simulink model "WindTurbineModelFinalPMSGASTW1"  (R2024a)
settings: Solver=ode1  StartTime=0.0  StopTime=50  FixedStep=0.0001  RelTol=1e-3
InitFcn:
  | ng       = 97;
model workspace: external: MAT-File C:\Users\anif4\Downloads\Cp_Model_5thOrder.mat (data not in the file)
settings Model: Creator=user  LastModifiedBy=anif4
settings RTWCC: GPUComputeCapability=3.5

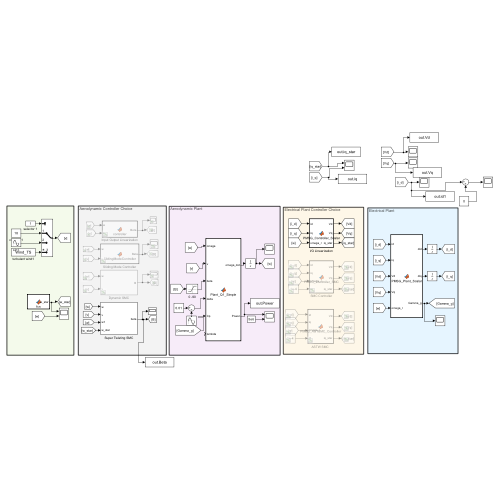
[thumbnail: Simulink's stored preview of the top-level diagram]
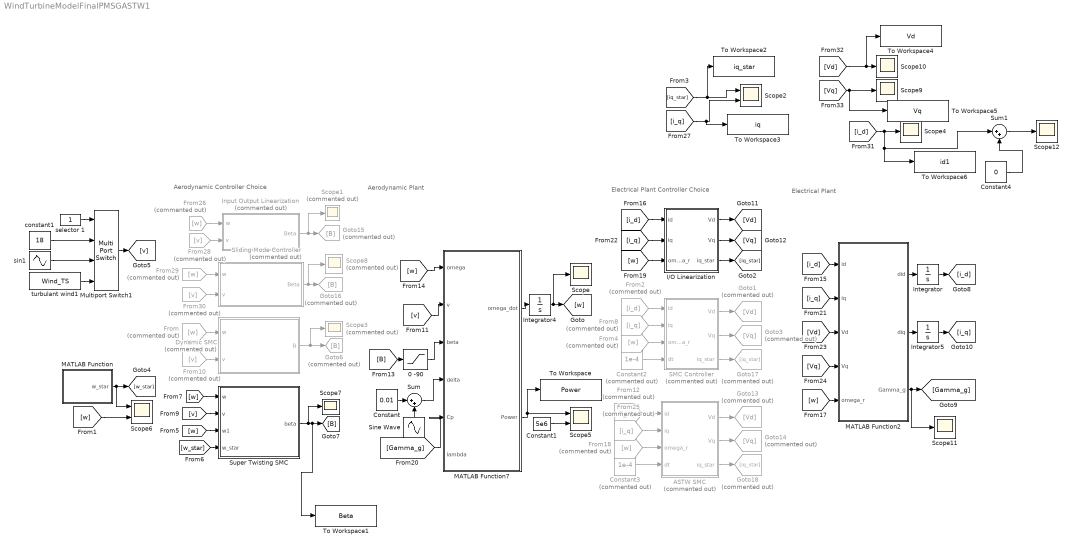
== system WindTurbineModelFinalPMSGASTW1 ==
  note: Electrical Plant
  note: Electrical Plant Controller Choice
  note: Aerodynamic Controller Choice
  note: Aerodynamic Plant
  0 -90 : Saturate  UpperLimit=90  LowerLimit=0
  "ASTW SMC " : MATLAB Function  Commented=on  TreatAsAtomicUnit=on
  Constant : Constant  Value=0.01
  Constant1 : Constant  Value=5e6
  Constant2 : Constant  Commented=on  Value=1e-4
  Constant3 : Constant  Commented=on  Value=1e-4
  Constant4 : Constant  Value=0
  Dynamic SMC : Subsystem  Commented=on
  From{,4,18,26,29} (5 alike) : From  Commented=on  GotoTag=w
  From10 : From  Commented=on  GotoTag=v
  From12 : From  Commented=on  GotoTag=i_d
  From2 : From  Commented=on  GotoTag=i_d
  From25 : From  Commented=on  GotoTag=i_q
  From28 : From  Commented=on  GotoTag=v
  From30 : From  Commented=on  GotoTag=v
  From8 : From  Commented=on  GotoTag=i_q
  Goto1 : Goto  Commented=on  GotoTag=Vd
  Goto13 : Goto  Commented=on  GotoTag=Vd
  Goto14 : Goto  Commented=on  GotoTag=Vq
  Goto15 : Goto  Commented=on  GotoTag=B
  Goto16 : Goto  Commented=on  GotoTag=B
  Goto17 : Goto  Commented=on  GotoTag=iq_star
  Goto18 : Goto  Commented=on  GotoTag=iq_star
  Goto3 : Goto  Commented=on  GotoTag=Vq
  Goto6 : Goto  Commented=on  GotoTag=B
  I/O Linearization : MATLAB Function  TreatAsAtomicUnit=on
  Input Output Linearization : MATLAB Function  Commented=on  TreatAsAtomicUnit=on
  Integrator : Integrator
  Integrator4 : Integrator  InitialCondition=2
  Integrator5 : Integrator
  MATLAB Function : MATLAB Function  TreatAsAtomicUnit=on
  MATLAB Function2 : MATLAB Function  TreatAsAtomicUnit=on
  MATLAB Function7 : MATLAB Function  TreatAsAtomicUnit=on
  Multiport Switch1 : MultiPortSwitch  SaturateOnIntegerOverflow=off  InputSameDT=off
  SMC Controller : MATLAB Function  Commented=on  TreatAsAtomicUnit=on
  Scope{,4,7,9..12} (7 alike) : Scope
  Scope1 : Scope  Commented=on
  Scope2 : Scope  NumInputPorts=2
  Scope3 : Scope  Commented=on
  Scope5 : Scope  NumInputPorts=2
  Scope6 : Scope  NumInputPorts=2
  Scope8 : Scope  Commented=on
  Sine Wave : Sin  Amplitude=0.2  Frequency=0.5  SampleTime=0
  Sliding Mode Controller : MATLAB Function  Commented=on  TreatAsAtomicUnit=on
  Sum : Sum  Inputs=|++
  Sum1 : Sum  Inputs=|++
  Super Twisting SMC : Subsystem
  To Workspace : ToWorkspace  VariableName=Power  SampleTime=-1
  To Workspace1 : ToWorkspace  VariableName=Beta  SampleTime=-1
  To Workspace2 : ToWorkspace  VariableName=iq_star  SampleTime=-1
  To Workspace3 : ToWorkspace  VariableName=iq  SampleTime=-1
  To Workspace4 : ToWorkspace  VariableName=Vd  SampleTime=-1
  To Workspace5 : ToWorkspace  VariableName=Vq  SampleTime=-1
  To Workspace6 : ToWorkspace  VariableName=id1  SampleTime=-1
  constant1 : Constant  Value=18
  selector 1 : Constant
  sin1 : Sin  Bias=20  Frequency=0.5  SampleTime=0
  turbulant wind1 : FromWorkspace  VariableName=Wind_TS
  wires:
  selector 1/1 -> Multiport Switch1/1
  constant1/1 -> Multiport Switch1/2
  sin1/1 -> Multiport Switch1/3
  Multiport Switch1/1 -> [v]
  MATLAB Function7/2(Power) -> To Workspace/1, Scope5/1
  turbulant wind1/1 -> Multiport Switch1/4
  MATLAB Function7/1(omega_dot) -> Integrator4/1
  Constant1/1 -> Scope5/2
  Integrator4/1 -> [w], Scope/1
  Sum/1 -> MATLAB Function7/4(delta)
  Constant/1 -> Sum/1
  Sine Wave/1 -> Sum/2
  MATLAB Function/1(w_star) -> Scope6/1, [w_star]
  [w] -> Scope6/2
  0 -90/1 -> MATLAB Function7/3(beta)
  [v] -> MATLAB Function7/2(v)
  [B] -> 0 -90/1
  [w] -> MATLAB Function7/1(omega)
  [w] -> Super Twisting SMC/1(w)
  [v] -> Super Twisting SMC/2(v)
  [w] -> Super Twisting SMC/3(w1)
  [w_star] -> Super Twisting SMC/4(w_star)
  Super Twisting SMC/1(beta) -> To Workspace1/1, [B], Scope7/1
  From/1 -> Dynamic SMC/1(w)
  From10/1 -> Dynamic SMC/2(v)
  Dynamic SMC/1(B) -> Scope3/1, Goto6/1
  MATLAB Function2/1(did) -> Integrator/1
  Integrator/1 -> [i_d]
  [i_d] -> MATLAB Function2/1(id)
  [i_d] -> I/O Linearization/1(id)
  [w] -> MATLAB Function2/5(omega_r)
  [w] -> I/O Linearization/3(omega_r)
  MATLAB Function2/3(Gamma_g) -> Scope11/1, [Gamma_g]
  [Gamma_g] -> MATLAB Function7/5(Cp)
  Integrator5/1 -> [i_q]
  MATLAB Function2/2(diq) -> Integrator5/1
  [i_q] -> MATLAB Function2/2(iq)
  [i_q] -> I/O Linearization/2(iq)
  [Vd] -> MATLAB Function2/3(Vd)
  I/O Linearization/1(Vd) -> [Vd]
  [Vq] -> MATLAB Function2/4(Vq)
  I/O Linearization/2(Vq) -> [Vq]
  SMC Controller/1(Vd) -> Goto1/1
  SMC Controller/2(Vq) -> Goto3/1
  From2/1 -> SMC Controller/1(id)
  From8/1 -> SMC Controller/2(iq)
  From4/1 -> SMC Controller/3(omega_r)
  Constant2/1 -> SMC Controller/4(dt)
  From12/1 -> "ASTW SMC "/1(id)
  From25/1 -> "ASTW SMC "/2(iq)
  From18/1 -> "ASTW SMC "/3(omega_r)
  "ASTW SMC "/1(Vd) -> Goto13/1
  "ASTW SMC "/2(Vq) -> Goto14/1
  Constant3/1 -> "ASTW SMC "/4(dt)
  From29/1 -> Sliding Mode Controller/1(w)
  From30/1 -> Sliding Mode Controller/2(v)
  Sliding Mode Controller/1(Beta) -> Scope8/1, Goto16/1
  Input Output Linearization/1(Beta) -> Scope1/1, Goto15/1
  From28/1 -> Input Output Linearization/2(v)
  From26/1 -> Input Output Linearization/1(w)
  I/O Linearization/3(iq_star) -> [iq_star]
  [iq_star] -> To Workspace2/1, Scope2/1
  [i_d] -> Sum1/1, To Workspace6/1, Scope4/1
  [Vq] -> To Workspace5/1, Scope9/1
  [Vd] -> To Workspace4/1, Scope10/1
  [i_q] -> To Workspace3/1, Scope2/2
  SMC Controller/3(iq_star) -> Goto17/1
  "ASTW SMC "/3(iq_star) -> Goto18/1
  Constant4/1 -> Sum1/2
  Sum1/1 -> Scope12/1

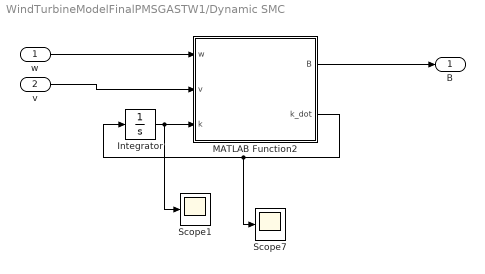
== system WindTurbineModelFinalPMSGASTW1/Dynamic SMC ==
  w : Inport
  v : Inport  Port=2
  Integrator : Integrator
  MATLAB Function2 : MATLAB Function  TreatAsAtomicUnit=on
  Scope1 : Scope
  Scope7 : Scope
  B : Outport
  wires:
  Integrator/1 -> MATLAB Function2/3(k), Scope1/1
  MATLAB Function2/2(k_dot) -> Scope7/1, Integrator/1
  w/1 -> MATLAB Function2/1(w)
  MATLAB Function2/1(B) -> B/1
  v/1 -> MATLAB Function2/2(v)

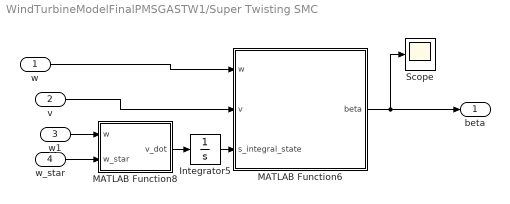
== system WindTurbineModelFinalPMSGASTW1/Super Twisting SMC ==
  w : Inport
  v : Inport  Port=2
  w1 : Inport  Port=3
  w_star : Inport  Port=4
  Integrator5 : Integrator
  MATLAB Function6 : MATLAB Function  TreatAsAtomicUnit=on
  MATLAB Function8 : MATLAB Function  TreatAsAtomicUnit=on
  Scope : Scope
  beta : Outport
  wires:
  MATLAB Function8/1(v_dot) -> Integrator5/1
  Integrator5/1 -> MATLAB Function6/3(s_integral_state)
  w/1 -> MATLAB Function6/1(w)
  w_star/1 -> MATLAB Function8/2(w_star)
  w1/1 -> MATLAB Function8/1(w)
  MATLAB Function6/1(beta) -> Scope/1, beta/1
  v/1 -> MATLAB Function6/2(v)

== matlab function WindTurbineModelFinalPMSGASTW1/SMC Controller ==
  settings: updateMethod=DISCRETE
  data: id input; Vd output; iq input; omega_r input; Vq output; dt input; iq_star output
function [Vd, Vq, iq_star] = PMSG_Controller_SMC(id, iq, omega_r, dt)
% Parameters
Rs =  1.06;         
Ld = 0.01429;      
Lq = 0.01429;  
phi_f = 8.6; 
p = 5; 
ng = 97;
P_star = 5e6; 

% Generator Dynamics
omega_g = ng * omega_r;
omega_e = p * omega_g;

% Persistent variables for the ST-SMC integral terms
persistent u_int_d u_int_q
if isempty(u_int_d)
    u_int_d = 0; u_int_q = 0;
end

%% 1. References
id_star = 0;
iq_star = (2 * P_star) / (3 * p * phi_f * ng * omega_r);

%% 2. Sliding Surfaces
sigma_d = id - id_star;
sigma_q = iq - iq_star;

%% 3. Super-Twisting Gains
% These gains should be tuned. k2 must be large enough to overcome 
% the derivative of the disturbances.
k1 = 500; 
k2 = 3500;

%% 4. SMC Control Law
% d-axis
u_int_d = u_int_d + (-k2 * sign(sigma_d)) * dt;
u_d = -k1 * sqrt(abs(sigma_d)) * sign(sigma_d) + u_int_d;

% q-axis
u_int_q = u_int_q + (-k2 * sign(sigma_q)) * dt;
u_q = -k1 * sqrt(abs(sigma_q)) * sign(sigma_q) + u_int_q;

%% 5. Feedback Linearization (Voltage Mapping)
% We use the SMC outputs to drive the Vd and Vq
Vd = Ld * u_d - omega_e * Lq * iq + Rs * id;
Vq = Lq * u_q + omega_e * Ld * id + omega_e * phi_f + Rs * iq;

end

== matlab function WindTurbineModelFinalPMSGASTW1/ASTW SMC  ==
  settings: updateMethod=DISCRETE
  data: id input; Vd output; iq input; omega_r input; Vq output; dt input; iq_star output
function [Vd, Vq, iq_star] = PMSG_ASTSMC_Controller(id, iq, omega_r, dt)
% --- Persistent Variables ---
persistent u_int_d u_int_q k1 k2 sigma_d_prev sigma_q_prev
if isempty(u_int_d)
    u_int_d = 0; u_int_q = 0; k1 = 50; k2 = 100; % Higher initial values
    sigma_d_prev = 0; sigma_q_prev = 0;
end

% --- Parameters ---
Rs = 0.53; Ld = 0.01429; Lq = 0.01429; phi_f = 8.6; p = 5; ng = 97; P_star = 5e6;
omega_e = p * ng * omega_r;

% --- 1. Sliding Surfaces ---
id_star = 0;
iq_star = (2 * P_star) / (3 * p * phi_f * ng * omega_r);
sigma_d = id - id_star;
sigma_q = iq - iq_star;

% --- 2. Adaptive Gain Dynamics (Improved Algorithm 3/4) ---
alpha0 = 2000;  % Base adaptation speed (Increase this if tracking is slow)
epsilon = 0.5;  % Larger boundary layer to prevent premature gain decay

% Psi = -dot(sigma)
psi_q = -(sigma_q - sigma_q_prev) / dt;
sigma_q_prev = sigma_q;

% Adaptation logic for k1 and k2
if abs(sigma_q) > epsilon
    % Increase gains according to the documentation
    dk1 = alpha0 / (abs(psi_q) + 0.01); 
    dk2 = alpha0 / (2 * sqrt(abs(sigma_q)));
else
    % Use a CONSTANT decay rate instead of -k1. 
    % This stops the gains from dropping to zero.
    dk1 = -10; 
    dk2 = -50; 
end

% Update and protect gains (Ensure they stay above a functional minimum)
k1 = max(k1 + dk1 * dt, 1000); 
k2 = max(k2 + dk2 * dt, 1500);

% --- 3. Super-Twisting Control Law ---
u_int_d = u_int_d + (-k2 * sign(sigma_d)) * dt;
u_d = -k1 * sqrt(abs(sigma_d)) * sign(sigma_d) + u_int_d;

u_int_q = u_int_q + (-k2 * sign(sigma_q)) * dt;
u_q = -k1 * sqrt(abs(sigma_q)) * sign(sigma_q) + u_int_q;

% --- 4. Final Control Voltages ---
Vd = Ld * u_d - omega_e * Lq * iq + Rs * id;
Vq = Lq * u_q + omega_e * Ld * id + omega_e * phi_f + Rs * iq;
end

== matlab function WindTurbineModelFinalPMSGASTW1/Sliding Mode Controller ==
  data: w input; Beta output; v input
function Beta  = SlidingModeController(w,v)

% Parameters
ng       = 97;
taugStar = 43093;      % N.m (generator rated torque)
R        = 63;         % m
rho      = 1.22;       % kg/m^3
J        = 38759228;   % kg.m^2

% Tip-speed ratio
lambda = (w * R) / v;  
k=10;
% Coefficients
c0 = 0.5;  c1 = 73.5; c2 = 0.4; c3 = 5;
c4 = 13.125; c5 = 0.08; c6 = 0.035;
u=20;
% Aerodynamic Cp approximation (depends on lambda and beta)
lambda1_inv = 1/(lambda + c5*u) - c6/(u^3 + 1);
a = -(c0*c2) * exp(-c4*lambda1_inv);
b =  (c0*(c1*lambda1_inv - c3)) * exp(-c4*lambda1_inv);
Cp = a*u + b;      % Cp in affine-form w.r.t. beta
Cp = min(max(Cp, 0), 0.5);

n_g=97; %Gearbox ratio
t_g=4.309355*10^4;  %Rated generator torque
P_star=5*10^6; % Rated electrical power

w_star=P_star/(n_g*t_g);
s = w - w_star;
%e_dot=-k*e;
F = (1/J) * ( ((0.5 * rho * pi * R^3 * v^2)/lambda)*b - ng*taugStar );
G = (1/J) * ( ((0.5 * rho * pi * R^3 * v^2)/lambda)*a );

Beta= -(F/G)-(k*sign(s))/G;

end

== matlab function WindTurbineModelFinalPMSGASTW1/Dynamic SMC/MATLAB Function2 ==
  data: w input; B output; v input; k_dot output; k input
function [B,k_dot]  = DynamicGain_SlidingModeController(w,v,k)

% Parameters
ng       = 97;
taugStar = 43093;      % N.m (generator rated torque)
R        = 63;         % m
rho      = 1.22;       % kg/m^3
J        = 38759228;   % kg.m^2
E= 0.0003;

% Tip-speed ratio
lambda = (w * R) / v;  

% Coefficients
c0 = 0.5;  c1 = 73.5; c2 = 0.4; c3 = 5;
c4 = 13.125; c5 = 0.08; c6 = 0.035;
u=20;
% Aerodynamic Cp approximation (depends on lambda and beta)
lambda1_inv = 1/(lambda + c5*u) - c6/(u^3 + 1);
a = -(c0*c2) * exp(-c4*lambda1_inv);
b =  (c0*(c1*lambda1_inv - c3)) * exp(-c4*lambda1_inv);
Cp = a*u + b;      % Cp in affine-form w.r.t. beta
Cp = min(max(Cp, 0), 0.5);

n_g=97; %Gearbox ratio
t_g=4.309355*10^4;  %Rated generator torque
P_star=5*10^6; % Rated electrical power

w_star=P_star/(n_g*t_g);
s = w - w_star;
k_dot=0.5* sign(abs(s)-E);

%e_dot=-k*e;
F = (1/J) * ( ((0.5 * rho * pi * R^3 * v^2)/lambda)*b - ng*taugStar );
G = (1/J) * ( ((0.5 * rho * pi * R^3 * v^2)/lambda)*a );

B= -(F/G)-(k*sign(s))/G;

end

== matlab function WindTurbineModelFinalPMSGASTW1/MATLAB Function7 ==
  data: omega input; omega_dot output; v input; beta input; Power output; delta input; Cp input; lambda input
function [omega_dot, Power] = Plant_Q1_Simple(omega, v, beta, delta, Cp, lambda)
% Parameters
ng       = 97;
taugStar = 43093;      % N.m (generator rated torque)
R        = 63;         % m
rho      = 1.22;       % kg/m^3
J        = 38759228;   % kg.m^2

% --- REMOVED INTERNAL CALCULATIONS ---
% Internal lambda and Cp calculations are removed because they are now
% passed in as arguments from the Simulink model.

% Coefficients needed for F and G terms
c0 = 0.5;  c1 = 73.5; c2 = 0.4; c3 = 5;
c4 = 13.125; c5 = 0.08; c6 = 0.035;
u = beta; 

% We still need the 'a' and 'b' components to calculate omega_dot 
% in the affine form (F + G*u), using the external lambda.
lambda1_inv = 1/(lambda + c5*u) - c6/(u^3 + 1);
a = -(c0*c2) * exp(-c4*lambda1_inv);
b =  (c0*(c1*lambda1_inv - c3)) * exp(-c4*lambda1_inv);

% Power calculation
Power = taugStar * ng * omega ;   % Aerodynamic power

% ---- F + G*u form ----
% Note: This uses the 'a' and 'b' derived from the external lambda
F = (1/J) * ( ((0.5 * rho * pi * R^3 * v^2)/omega)*b - ng*taugStar );
G = (1/J) * ( ((0.5 * rho * pi * R^3 * v^2)/omega)*a );

omega_dot = F + G*u + delta;

end

== matlab function WindTurbineModelFinalPMSGASTW1/MATLAB Function ==
  data: w_star output
function w_star = fcn()
ng       = 97;
taugStar = 43093;      % N.m (generator rated torque)
R        = 63;         % m
rho      = 1.22;       % kg/m^3
J        = 38759228;

n_g=97; %Gearbox ratio
t_g=4.309355*10^4;  %Rated generator torque
P_star=5*10^6; % Rated electrical power

w_star=P_star/(n_g*t_g);

== matlab function WindTurbineModelFinalPMSGASTW1/Input Output Linearization ==
  data: w input; Beta output; v input
function Beta  = controller(w,v)

% Parameters
ng       = 97;
taugStar = 43093;      % N.m (generator rated torque)
R        = 63;         % m
rho      = 1.22;       % kg/m^3
J        = 38759228;   % kg.m^2

% Tip-speed ratio
lambda = (w * R) / v;  
k=45;
% Coefficients
c0 = 0.5;  c1 = 73.5; c2 = 0.4; c3 = 5;
c4 = 13.125; c5 = 0.08; c6 = 0.035;
u=20;
% Aerodynamic Cp approximation (depends on lambda and beta)
lambda1_inv = 1/(lambda + c5*u) - c6/(u^3 + 1);
a = -(c0*c2) * exp(-c4*lambda1_inv);
b =  (c0*(c1*lambda1_inv - c3)) * exp(-c4*lambda1_inv);
Cp = a*u + b;      % Cp in affine-form w.r.t. beta
Cp = min(max(Cp, 0), 0.5);

n_g=97; %Gearbox ratio
t_g=4.309355*10^4;  %Rated generator torque
P_star=5*10^6; % Rated electrical power

w_star=P_star/(n_g*t_g);
e = w - w_star;
e_dot=-k*e;
F = (1/J) * ( ((0.5 * rho * pi * R^3 * v^2)/lambda)*b - ng*taugStar );
G = (1/J) * ( ((0.5 * rho * pi * R^3 * v^2)/lambda)*a );

Beta= (-F+e_dot)/G;

end

== matlab function WindTurbineModelFinalPMSGASTW1/Super Twisting SMC/MATLAB Function6 ==
  data: w input; beta output; v input; s_integral_state input
function beta  = SuperTwisting_Controller(w, v, s_integral_state)
% Parameters (matching your existing plant)
ng       = 97;
taugStar = 43093;      
R        = 63;         
rho      = 1.22;       
J        = 38759228;   
P_star   = 5e6;

% Calculate rated speed and sliding surface
w_star = P_star / (ng * taugStar);
s = w - w_star;

% --- Gains Selection ---
% Tune k1 and k2 based on the bound of your perturbation delta(t)
k1 = 0.6; 
k2 = 0.05;

% --- Plant Dynamics (F and G) ---
lambda = (w * R) / v;
c0 = 0.5; c1 = 73.5; c2 = 0.4; c3 = 5;
c4 = 13.125; c5 = 0.08; c6 = 0.035;

% For linearization, we use a nominal pitch (e.g., u = 20)
u_nom = 20; 
lambda1_inv = 1/(lambda + c5*u_nom) - c6/(u_nom^3 + 1);
a = -(c0*c2) * exp(-c4*lambda1_inv);
b = (c0*(c1*lambda1_inv - c3)) * exp(-c4*lambda1_inv);

F = (1/J) * ( ((0.5 * rho * pi * R^3 * v^2)/lambda)*b - ng*taugStar );
G = (1/J) * ( ((0.5 * rho * pi * R^3 * v^2)/lambda)*a );

% --- Super-Twisting Law ---
% u_sta = -k1 * |s|^0.5 * sign(s) + v_dot_integral
u_sta = -k1 * sqrt(abs(s)) * sign(s) + s_integral_state;

beta = (u_sta - F) / G;
end

== matlab function WindTurbineModelFinalPMSGASTW1/Super Twisting SMC/MATLAB Function8 ==
  data: w input; v_dot output; w_star input
function v_dot = fcn(w, w_star)
k2 = 0.02;
s = w - w_star;

v_dot = -k2*sign(s);


end

== matlab function WindTurbineModelFinalPMSGASTW1/MATLAB Function2 ==
  data: id input; did output; diq output; iq input; Vd input; Vq input; omega_r input; Gamma_g output
function [did, diq, Gamma_g] = PMSG_Plant_Scalar(id, iq, Vd, Vq, omega_r)
% Parameters [cite: 98]
Rs = 1.06;         
Ld = 0.01429;      
Lq =  0.01429;      
phi_f = 8.6;       
p = 5;             
ng = 97;           

% Generator speed [cite: 63]
omega_g = ng * omega_r; 

% Electrical differential equations [cite: 62]
did = (-Rs/Ld)*id + (p*Lq/Ld)*omega_g*iq + (1/Ld)*Vd;
diq = (-Rs/Lq)*iq - (p*Ld/Lq)*omega_g*id - (p*phi_f/Lq)*omega_g + (1/Lq)*Vq;

Gamma_g = (3/2)*p*phi_f*iq;
end

== matlab function WindTurbineModelFinalPMSGASTW1/I//O Linearization ==
  data: id input; iq input; Vd output; omega_r input; Vq output; iq_star output
function [Vd, Vq, iq_star] = PMSG_Controller_Scalar(id, iq, omega_r)
% Parameters
Rs = 1.06;         
Ld =  0.01429;      
Lq =  0.01429;  
phi_f = 8.6; 
p = 5; 
ng = 97;
P_star = 5e6; % Rated Power 5MW 

% Generator speed calculation 
omega_g = ng * omega_r;

% Define References [cite: 67, 79]
id_star = 0;
iq_star = (2 * P_star) / (3 * ng * omega_r * p * phi_f);

% Error Dynamics Gains (Start with 500, adjust if slow)
lambda_i = 500; 
u_d = -lambda_i * (id - id_star);
u_q = -lambda_i * (iq - iq_star);

% 3. Control Law (Input-Output Linearization)
Vd = Ld * (u_d + (Rs/Ld)*id - (p*Lq/Ld)*omega_g*iq);
Vq = Lq * (u_q + (Rs/Lq)*iq + (p*Ld/Lq)*omega_g*id + (p*phi_f/Lq)*omega_g);
end
